simulink model "innerLoop_currentControl"  (R2024a)
settings: Solver=FixedStepAuto  StartTime=0.0  StopTime=Tsim_inLoop  FixedStep=Tsw  RelTol=1e-3
undefined symbols (not defined in the file): den_aaf, den_i, DiscIntNeverNeededParam, ILnom, kaw_i, ki_i, kp_i, kpf_i, L, num_aaf, num_i, RserL, Tsim_inLoop, Tsw, VinNom, VLlim, VoutNom, zden_aaf, zden_pf_i, zden_plant_i, znum_aaf, znum_pf_i, znum_plant_i
libraries: simulink x5
settings Model: Creator=nicholas  LastModifiedBy=nicholas
settings RTWCC: GPUComputeCapability=3.5

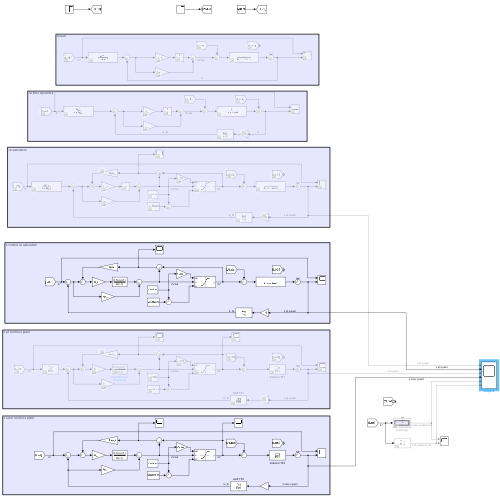
[thumbnail: Simulink's stored preview of the top-level diagram]
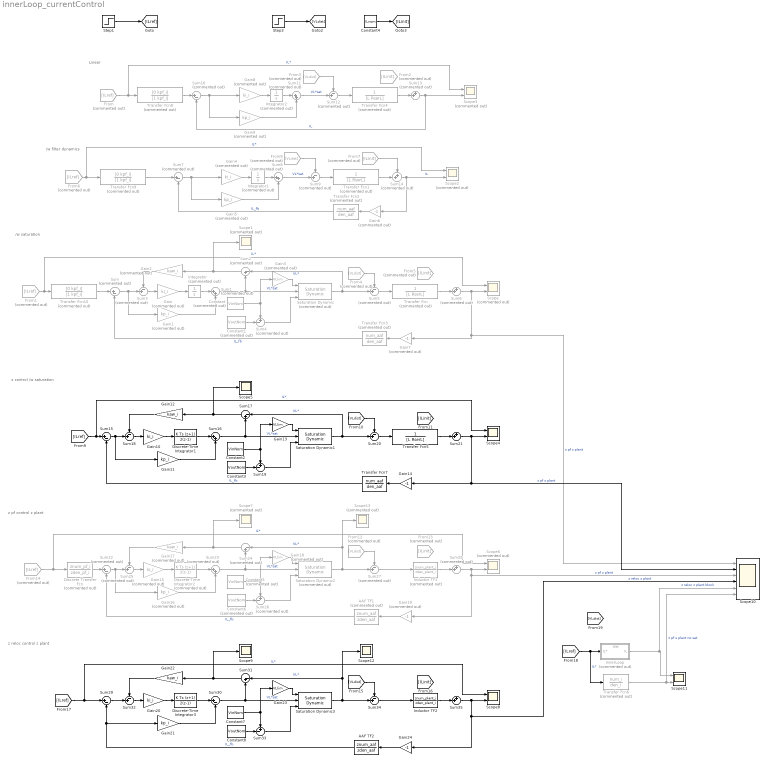
== system innerLoop_currentControl ==
  note: /w saturation
  note: /w filter dynamics
  note: Linear
  note: z control /w saturation
  note: z pf control z plant
  note: z reloc control z plant
  AAF TF1 : DiscreteTransferFcn  Commented=on  Numerator=znum_aaf  Denominator=zden_aaf
  AAF TF2 : DiscreteTransferFcn  Numerator=znum_aaf  Denominator=zden_aaf
  Constant : Constant  Commented=on  Value=VinNom
  Constant1 : Constant  Commented=on  Value=VoutNom
  Constant2 : Constant  Value=VinNom
  Constant3 : Constant  Value=VoutNom
  Constant4 : Constant  Value=ILnom  SampleTime=-1
  Constant5 : Constant  Commented=on  Value=VinNom
  Constant6 : Constant  Commented=on  Value=VoutNom
  Constant7 : Constant  Value=VinNom
  Constant8 : Constant  Value=VoutNom
  Discrete Transfer Fcn : DiscreteTransferFcn  Commented=on  Numerator=znum_pf_i  Denominator=zden_pf_i
  Discrete-Time Integrator1 : DiscreteIntegrator  IntegratorMethod=Integration: Trapezoidal  SampleTime=Tsw  ICPrevOutput=DiscIntNeverNeededParam  ICPrevScaledInput=DiscIntNeverNeededParam
  Discrete-Time Integrator2 : DiscreteIntegrator  Commented=on  IntegratorMethod=Integration: Trapezoidal  SampleTime=Tsw  ICPrevOutput=DiscIntNeverNeededParam  ICPrevScaledInput=DiscIntNeverNeededParam
  Discrete-Time Integrator3 : DiscreteIntegrator  IntegratorMethod=Integration: Trapezoidal  SampleTime=Tsw  ICPrevOutput=DiscIntNeverNeededParam  ICPrevScaledInput=DiscIntNeverNeededParam
  From{,1,6,14} (4 alike) : From  Commented=on  GotoTag=ILref
  From{3..4,8,12} (4 alike) : From  Commented=on  GotoTag=VLdist
  From{2,5,7,13} (4 alike) : From  Commented=on  GotoTag=ILinit
  Gain{,4,8,15} (4 alike) : Gain  Commented=on  Gain=ki_i
  Gain{1,5,9,16} (4 alike) : Gain  Commented=on  Gain=kp_i
  Gain10 : Gain  Gain=ki_i
  Gain11 : Gain  Gain=kp_i
  Gain12 : Gain  Gain=kaw_i
  Gain13 : Gain  Gain=VLlim
  Gain14 : Gain  Gain=-1
  Gain17 : Gain  Commented=on  Gain=kaw_i
  Gain18 : Gain  Commented=on  Gain=VLlim
  Gain19 : Gain  Commented=on  Gain=-1
  Gain2 : Gain  Commented=on  Gain=kaw_i
  Gain20 : Gain  Gain=ki_i
  Gain21 : Gain  Gain=kp_i
  Gain22 : Gain  Gain=kaw_i
  Gain23 : Gain  Gain=VLlim
  Gain24 : Gain  Gain=-1
  Gain3 : Gain  Commented=on  Gain=VLlim
  Gain6 : Gain  Commented=on  Gain=-1
  Gain7 : Gain  Commented=on  Gain=-1
  Inductor TF1 : DiscreteTransferFcn  Commented=on  Numerator=znum_plant_i  Denominator=zden_plant_i
  Inductor TF2 : DiscreteTransferFcn  Numerator=znum_plant_i  Denominator=zden_plant_i
  InnerLoop : Subsystem  Commented=on
      settings: PortSchema="{\"entries\":[{\"content\":{\"sides\":[{\"content\":{\"connectorIds\":[\"In1\"]},\"type\":\"ConnectorPlacement.EquallySpacedRectSide\",\"uuid\":\"ea8557f0-2829-4e37-b4b3-547e1edede5f\"},{\"content\":{\"connectorIds\":[\"Out1\"],\"side\":\"RIGHT\"},\"type\":\"ConnectorPlacement.EquallySpacedRectSide\",\"uuid\":\"1f5eaae7-1846-4e2b-9076-d6e50ab32c3c\"},{\"content\":{\"connectorIds\":[\"In2\"],\"side\":\"TOP\"},\"type\":\"ConnectorPlacement.EquallySpacedRectSide\",\"uuid\":\"2796d338-5137-4815-8d3b-5e9fd8d8ca19\"},{\"content\":{\"side\":\"BOTTOM\"},\"type\":\"ConnectorPlacement.EquallySpacedRectSide\",\"uuid\":\"fc25d8da-de45-48fe-93ad-4a8a015fa227\"}]},\"type\":\"ConnectorPlacement.EquallySpacedConnector\",\"uuid\":\"235e4e93-e51a-4d68-867a-75744b50ca49\"}],\"packageUris\":[\"http://schema.mathworks.com/mf0/Connector/R2020b\"],\"version\":\"1.0\"}"
  Integrator : Integrator  Commented=on
  Integrator1 : Integrator  Commented=on
  Integrator2 : Integrator  Commented=on
  Saturation Dynamic : simulink/Discontinuities/Saturation Dynamic  Commented=on  OutMin=[]  OutMax=[]  OutDataTypeStr=Inherit: Same as second input  OutDataType=fixdt(1, 16)  OutScaling=2^-10  DoSatur=off
  Saturation Dynamic1 : simulink/Discontinuities/Saturation Dynamic  OutMin=[]  OutMax=[]  OutDataTypeStr=Inherit: Same as second input  OutDataType=fixdt(1, 16)  OutScaling=2^-10  DoSatur=off
  Saturation Dynamic2 : simulink/Discontinuities/Saturation Dynamic  Commented=on  OutMin=[]  OutMax=[]  OutDataTypeStr=Inherit: Same as second input  OutDataType=fixdt(1, 16)  OutScaling=2^-10  DoSatur=off
  Saturation Dynamic3 : simulink/Discontinuities/Saturation Dynamic  OutMin=[]  OutMax=[]  OutDataTypeStr=Inherit: Same as second input  OutDataType=fixdt(1, 16)  OutScaling=2^-10  DoSatur=off
  Scope{,2..3,6} (4 alike) : Scope  Commented=on  NumInputPorts=2
  Scope1 : Scope  Commented=on
  Scope10 : Scope  NumInputPorts=6
  Scope11 : Scope  NumInputPorts=2
  Scope12 : Scope
  Scope13 : Scope  Commented=on
  Scope4 : Scope  NumInputPorts=2
  Scope5 : Scope
  Scope7 : Scope  Commented=on
  Scope8 : Scope  NumInputPorts=2
  Scope9 : Scope
  Step1 : Step  Time=Tsim_inLoop/4  After=ILnom
  Step3 : Step  Time=Tsim_inLoop/2  After=VinNom/4
  Sum{,7,10,22} (4 alike) : Sum  Commented=on  Inputs=|+-
  Sum{1,8,11,23} (4 alike) : Sum  Commented=on  Inputs=|++
  Sum{3,5,9,12,25,27} (6 alike) : Sum  Commented=on  Inputs=-+|
  Sum{6,13..14,28} (4 alike) : Sum  Commented=on  Inputs=++|
  Sum15 : Sum  Inputs=|+-
  Sum16 : Sum  Inputs=|++
  Sum17 : Sum  Inputs=|-+
  Sum{18,20,32,34} (4 alike) : Sum  Inputs=-+|
  Sum19 : Sum  Inputs=+-|
  Sum2 : Sum  Commented=on  Inputs=|-+
  Sum21 : Sum  Inputs=++|
  Sum24 : Sum  Commented=on  Inputs=|-+
  Sum26 : Sum  Commented=on  Inputs=+-|
  Sum29 : Sum  Inputs=|+-
  Sum30 : Sum  Inputs=|+-
  Sum31 : Sum  Inputs=|-+
  Sum33 : Sum  Inputs=+-|
  Sum35 : Sum  Inputs=++|
  Sum4 : Sum  Commented=on  Inputs=+-|
  Transfer Fcn : TransferFcn  Commented=on  Denominator=[L RserL]
  Transfer Fcn1 : TransferFcn  Commented=on  Denominator=[L RserL]
  Transfer Fcn10 : TransferFcn  Commented=on  Numerator=[0 kpf_i]  Denominator=[1 kpf_i]
  Transfer Fcn2 : TransferFcn  Commented=on  Numerator=num_aaf  Denominator=den_aaf
  Transfer Fcn3 : TransferFcn  Commented=on  Numerator=num_aaf  Denominator=den_aaf
  Transfer Fcn4 : TransferFcn  Commented=on  Denominator=[L RserL]
  Transfer Fcn5 : TransferFcn  Denominator=[L RserL]
  Transfer Fcn6 : TransferFcn  Commented=on  Numerator=num_i  Denominator=den_i
  Transfer Fcn7 : TransferFcn  Numerator=num_aaf  Denominator=den_aaf
  Transfer Fcn8 : TransferFcn  Commented=on  Numerator=[0 kpf_i]  Denominator=[1 kpf_i]
  Transfer Fcn9 : TransferFcn  Commented=on  Numerator=[0 kpf_i]  Denominator=[1 kpf_i]
  wires:
  Sum/1 -> Sum3/2, Gain1/1
  Gain/1 -> Integrator/1
  Integrator/1 -> Sum1/1
  Gain1/1 -> Sum1/2
  Sum1/1 -> Saturation Dynamic/2, Sum2/2  "VL*sat"
  Saturation Dynamic/1 -> Sum5/2, Sum2/1  "VL*"
  Sum3/1 -> Gain/1
  Gain2/1 -> Sum3/1
  Sum4/1 -> Saturation Dynamic/3
  Constant/1 -> Gain3/1, Sum4/1
  Constant1/1 -> Sum4/2
  Gain3/1 -> Saturation Dynamic/1
  Sum2/1 -> Scope1/1, Gain2/1
  From1/1 -> Scope/1, Transfer Fcn10/1  "IL*"
  From/1 -> Scope3/1, Transfer Fcn8/1  "IL*"
  Sum10/1 -> Gain8/1, Gain9/1
  Integrator2/1 -> Sum11/1
  Gain8/1 -> Integrator2/1
  Gain9/1 -> Sum11/2
  Sum11/1 -> Sum12/2  "VL*sat"
  Transfer Fcn4/1 -> Sum13/2
  Sum12/1 -> Transfer Fcn4/1
  Sum13/1 -> Sum10/2, Scope3/2  "IL"
  Step1/1 -> [ILref]
  From3/1 -> Sum12/1
  From4/1 -> Sum5/1
  Sum5/1 -> Transfer Fcn/1
  Transfer Fcn/1 -> Sum6/2
  Sum6/1 -> Scope/2, Scope10/1, Gain7/1  "s pf s plant"
  Constant4/1 -> [ILinit]
  Transfer Fcn1/1 -> Sum14/2
  Gain5/1 -> Sum8/2
  Integrator1/1 -> Sum8/1
  Sum9/1 -> Transfer Fcn1/1
  Sum8/1 -> Sum9/2  "VL*sat"
  Sum7/1 -> Gain4/1, Gain5/1
  From8/1 -> Sum9/1
  Gain4/1 -> Integrator1/1
  From6/1 -> Scope2/1, Transfer Fcn9/1  "IL*"
  Sum14/1 -> Gain6/1, Scope2/2  "IL"
  From7/1 -> Sum14/1
  Transfer Fcn2/1 -> Sum7/2  "IL_fb"
  Gain6/1 -> Transfer Fcn2/1
  Gain7/1 -> Transfer Fcn3/1
  Transfer Fcn3/1 -> Sum/2  "IL_fb"
  Sum19/1 -> Saturation Dynamic1/3
  Gain13/1 -> Saturation Dynamic1/1
  Constant2/1 -> Gain13/1, Sum19/1
  Gain10/1 -> Discrete-Time Integrator1/1
  Transfer Fcn5/1 -> Sum21/2
  Gain11/1 -> Sum16/2
  Constant3/1 -> Sum19/2
  Sum18/1 -> Gain10/1
  Gain12/1 -> Sum18/1
  [ILref] -> Scope4/1, Sum15/1  "IL*"
  Sum20/1 -> Transfer Fcn5/1
  Sum15/1 -> Gain11/1, Sum18/2
  Discrete-Time Integrator1/1 -> Sum16/1
  Sum17/1 -> Gain12/1, Scope5/1
  [VLdist] -> Sum20/1
  Saturation Dynamic1/1 -> Sum20/2, Sum17/1  "VL*"
  Gain14/1 -> Transfer Fcn7/1
  Transfer Fcn7/1 -> Sum15/2  "IL_fb"
  Sum16/1 -> Saturation Dynamic1/2, Sum17/2  "VL*sat"
  Sum21/1 -> Scope4/2, Scope10/2, Gain14/1  "z pf s plant"
  Gain19/1 -> AAF TF1/1
  Sum23/1 -> Saturation Dynamic2/2, Sum24/2  "VL*sat"
  Gain18/1 -> Saturation Dynamic2/1
  Sum26/1 -> Saturation Dynamic2/3
  Sum24/1 -> Gain17/1, Scope7/1
  Sum22/1 -> Gain16/1, Sum25/2
  Sum28/1 -> Scope6/2, Gain19/1, Scope10/3  "z pf z plant"
  Sum25/1 -> Gain15/1
  AAF TF1/1 -> Sum22/2  "IL_fb"
  Constant6/1 -> Sum26/2
  Gain17/1 -> Sum25/1
  Inductor TF1/1 -> Sum28/2
  Constant5/1 -> Gain18/1, Sum26/1
  Sum27/1 -> Inductor TF1/1
  Discrete-Time Integrator2/1 -> Sum23/1
  Gain15/1 -> Discrete-Time Integrator2/1
  Gain16/1 -> Sum23/2
  From14/1 -> Scope6/1, Discrete Transfer Fcn/1  "IL*"
  Saturation Dynamic2/1 -> Sum27/2, Scope13/1, Sum24/1  "VL*"
  Discrete Transfer Fcn/1 -> Sum22/1
  Transfer Fcn8/1 -> Sum10/1
  Transfer Fcn9/1 -> Sum7/1
  Transfer Fcn10/1 -> Sum/1
  Sum32/1 -> Gain20/1
  Sum35/1 -> Scope8/2, Scope10/4, Gain24/1  "z reloc z plant"
  Gain24/1 -> AAF TF2/1
  AAF TF2/1 -> Gain21/1, Sum29/2  "IL_fb"
  Inductor TF2/1 -> Sum35/2
  Saturation Dynamic3/1 -> Scope12/1, Sum31/1, Sum34/2  "VL*"
  [ILref] -> Sum29/1, Scope8/1  "IL*"
  Gain21/1 -> Sum30/2
  Sum31/1 -> Gain22/1, Scope9/1
  Sum33/1 -> Saturation Dynamic3/3
  [VLdist] -> Sum34/1
  Sum30/1 -> Saturation Dynamic3/2, Sum31/2  "VL*sat"
  Gain20/1 -> Discrete-Time Integrator3/1
  Gain22/1 -> Sum32/1
  Constant8/1 -> Sum33/2
  Constant7/1 -> Gain23/1, Sum33/1
  Sum29/1 -> Sum32/2
  Sum34/1 -> Inductor TF2/1
  Discrete-Time Integrator3/1 -> Sum30/1
  Gain23/1 -> Saturation Dynamic3/1
  [ILref] -> Transfer Fcn6/1, InnerLoop/1(IL*)  "IL*"
  InnerLoop/1(IL) -> Scope10/5, Scope11/1  "z reloc z plant block"
  Transfer Fcn6/1 -> Scope10/6, Scope11/2  "z pf s plant no sat"
  Step3/1 -> [VLdist]
  From12/1 -> Sum27/1

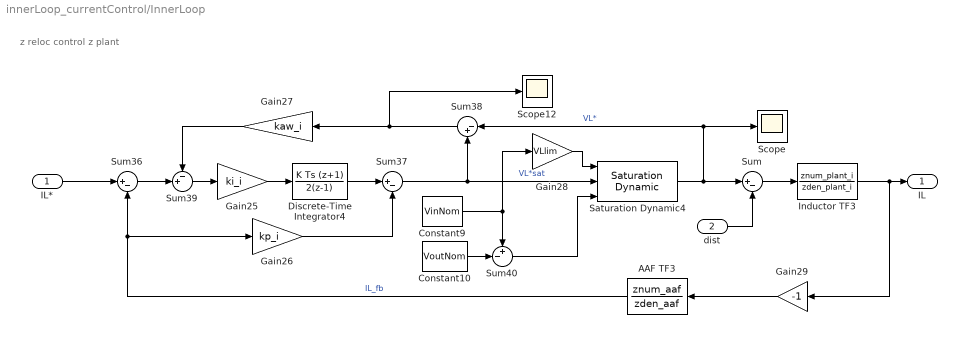
== system innerLoop_currentControl/InnerLoop ==
  note: z reloc control z plant
  IL* : Inport
  dist : Inport  Port=2
  AAF TF3 : DiscreteTransferFcn  Numerator=znum_aaf  Denominator=zden_aaf
  Constant10 : Constant  Value=VoutNom
  Constant9 : Constant  Value=VinNom
  Discrete-Time Integrator4 : DiscreteIntegrator  IntegratorMethod=Integration: Trapezoidal  SampleTime=Tsw  ICPrevOutput=DiscIntNeverNeededParam  ICPrevScaledInput=DiscIntNeverNeededParam
  Gain25 : Gain  Gain=ki_i
  Gain26 : Gain  Gain=kp_i
  Gain27 : Gain  Gain=kaw_i
  Gain28 : Gain  Gain=VLlim
  Gain29 : Gain  Gain=-1
  Inductor TF3 : DiscreteTransferFcn  Numerator=znum_plant_i  Denominator=zden_plant_i
  Saturation Dynamic4 : simulink/Discontinuities/Saturation Dynamic  OutMin=[]  OutMax=[]  OutDataTypeStr=Inherit: Same as second input  OutDataType=fixdt(1, 16)  OutScaling=2^-10  DoSatur=off
  Scope : Scope
  Scope12 : Scope
  Sum : Sum  Inputs=|+-
  Sum36 : Sum  Inputs=|+-
  Sum37 : Sum  Inputs=|+-
  Sum38 : Sum  Inputs=|-+
  Sum39 : Sum  Inputs=-+|
  Sum40 : Sum  Inputs=+-|
  IL : Outport
  wires:
  Sum40/1 -> Saturation Dynamic4/3
  Sum37/1 -> Saturation Dynamic4/2, Sum38/2  "VL*sat"
  Saturation Dynamic4/1 -> Sum/1, Scope/1, Sum38/1  "VL*"
  Sum38/1 -> Gain27/1, Scope12/1
  Sum39/1 -> Gain25/1
  Gain26/1 -> Sum37/2
  Constant10/1 -> Sum40/2
  Discrete-Time Integrator4/1 -> Sum37/1
  Inductor TF3/1 -> Gain29/1, IL/1
  Gain25/1 -> Discrete-Time Integrator4/1
  AAF TF3/1 -> Gain26/1, Sum36/2  "IL_fb"
  Gain29/1 -> AAF TF3/1
  Gain27/1 -> Sum39/1
  Constant9/1 -> Gain28/1, Sum40/1
  Sum36/1 -> Sum39/2
  Gain28/1 -> Saturation Dynamic4/1
  IL*/1 -> Sum36/1
  Sum/1 -> Inductor TF3/1
  dist/1 -> Sum/2
